simulink model "simple"  (Simulink 8.1)
settings: Solver=ode45  StartTime=0.0  StopTime=10.0  RelTol=1e-3
values from neighbouring files (symbols this model uses):
  g = 9.81    [parametry.m]
  l = 0.165    [parametry.m]
  m = 0.192    [parametry.m]
  M = 0.604    [parametry.m]
  theta0 = 0    [suwnica.m]
  thetaprim0 = 0.05    [suwnica.m]
  x0 = [x0 xprim0 theta0 thetaprim0]    [suwnica.m]
  xprim0 = 0    [suwnica.m]
libraries: simulink x1
settings Model: Creator=Michał  LastModifiedBy=Michał
settings DataIOCC: SignalLoggingSaveFormat=Dataset
settings OptimizationCC: ExpressionDepthLimit=128
settings DebuggingCC: FcnCallInpInsideContextMsg=EnableAllAsError
settings GRTTargetCC: CombineOutputUpdateFcns=on  GRTInterface=off

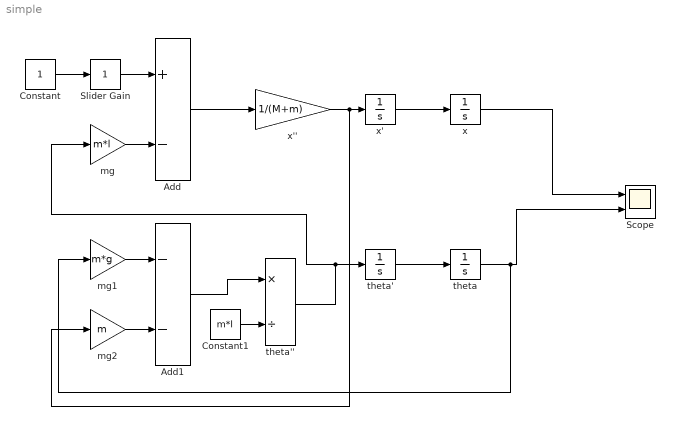
== system simple ==
  Add : Sum  Inputs=+-
  Add1 : Sum  Inputs=--
  Constant : Constant
  Constant1 : Constant  Value=m*l
  Scope : Scope  NumInputPorts=2
      settings: YMin=-5~-5  YMax=5~5
  Slider Gain : simulink/Math Operations/Slider Gain  low=-5  gain=1  high=5
  mg : Gain  Gain=m*l
  mg1 : Gain  Gain=m*g
  mg2 : Gain  Gain=m
  theta : Integrator  InitialCondition=theta0
  theta' : Integrator  InitialCondition=thetaprim0
  theta'' : Product  Inputs=*/
  x : Integrator  InitialCondition=x0
  x' : Integrator  InitialCondition=xprim0
  x'' : Gain  Gain=1/(M+m)
  wires:
  x'/1 -> x/1
  theta'/1 -> theta/1
  x''/1 -> mg2/1, x'/1
  Constant/1 -> Slider Gain/1
  Slider Gain/1 -> Add/1
  Add/1 -> x''/1
  mg/1 -> Add/2
  theta''/1 -> mg/1, theta'/1
  Add1/1 -> theta''/1
  Constant1/1 -> theta''/2
  x/1 -> Scope/1
  theta/1 -> mg1/1, Scope/2
  mg1/1 -> Add1/1
  mg2/1 -> Add1/2
